simulink subsystem "rss_FaltInfoMng"  (R2023a)
settings: Solver=VariableStepAuto  StartTime=0.0  StopTime=10.0  RelTol=1e-3
undefined symbols (not defined in the file): Cdbl_tiSlwTaskSmpTi, Gbol_enFaltInfoManClr_C, Gu16_ctFaltDiaComSdlCnt_C, Gu16_ctFaltDiaFstSdlCnt_C, Gu16_ctFaltDiaSlwSdlCnt_C, Gu16_stCtlDFPMSt_C
libraries: simulink x5
settings Model: Creator=xiaoqiang.yuan  LastModifiedBy=xiaoqiang.yuan

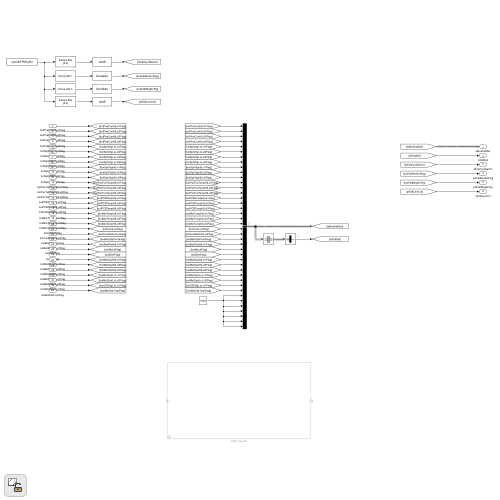
[thumbnail: Simulink's stored preview of the top-level diagram]
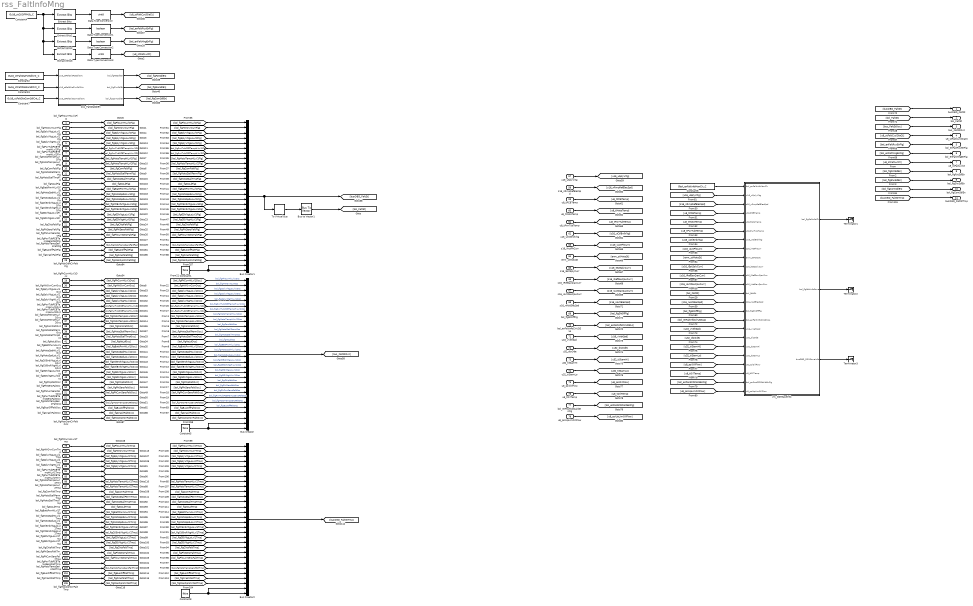
== system rss_FaltInfoMng ==
  bol_flgPhCurrHiLvl1Flg : Inport
  bol_flgHWOvrCurrFlg : Inport  Port=2
  bol_flgSplyVltgLoLvl1Flg : Inport  Port=3
  bol_flgSplyVltgLoLvl2Flg : Inport  Port=4
  bol_flgSplyVltgHiLvl1Flg : Inport  Port=5
  bol_flgPwrTubPCBTempHiLvl1Flg : Inport  Port=6
  bol_flgPwrTubPCBTempHiLvl2Flg : Inport  Port=7
  bol_flgMotoTempHiLvl1Flg : Inport  Port=8
  bol_flgMotoTempHiLvl2Flg : Inport  Port=9
  bol_flgComFaltFlg : Inport  Port=10
  bol_flgMotoStallPermFlg : Inport  Port=11
  bol_flgMotoStallTmpFlg : Inport  Port=12
  bol_flgNoLdFlg : Inport  Port=13
  bol_flgBattPwrHiLvl1Flg : Inport  Port=14
  bol_flgMotoSpdHiLvl1Flg : Inport  Port=15
  bol_flgMotoSpdLoLvl1Flg : Inport  Port=16
  bol_flgCtlBrdVltgLoLvl1Flg : Inport  Port=17
  bol_flgCtlBrdVltgHiLvl1Flg : Inport  Port=18
  bol_flgGDVltgLoLvl1Flg : Inport  Port=19
  bol_flgGDVltgHiLvl1Flg : Inport  Port=20
  bol_flgChipFaltFlg : Inport  Port=21
  bol_flgPhiSensFaltFlg : Inport  Port=22
  bol_flgPhCurrSensFaltFlg : Inport  Port=23
  bol_flgPwrTubPCBTempSensFaltFlg : Inport  Port=24
  bol_flgMotoTempSensFaltFlg : Inport  Port=25
  bol_flgBusOffFaltFlg : Inport  Port=26
  bol_flgCrashFaltFlg : Inport  Port=27
  bol_flgMosOpnCirFaltFlg : Inport  Port=28
  bol_flgPhCurrHiLvl1Occ : Inport  Port=29
  bol_flgHWOvrCurrOcc : Inport  Port=30
  bol_flgSplyVltgLoLvl1Occ : Inport  Port=31
  bol_flgSplyVltgLoLvl2Occ : Inport  Port=32
  bol_flgSplyVltgHiLvl1Occ : Inport  Port=33
  bol_flgPwrTubPCBTempHiLvl1Occ : Inport  Port=34
  bol_flgPwrTubPCBTempHiLvl2Occ : Inport  Port=35
  bol_flgMotoTempHiLvl1Occ : Inport  Port=36
  bol_flgMotoTempHiLvl2Occ : Inport  Port=37
  bol_flgComFaltOcc : Inport  Port=38
  bol_flgMotoStallPermOcc : Inport  Port=39
  bol_flgMotoStallTmpOcc : Inport  Port=40
  bol_flgNoLdOcc : Inport  Port=41
  bol_flgBattPwrHiLvl1Occ : Inport  Port=42
  bol_flgMotoSpdHiLvl1Occ : Inport  Port=43
  bol_flgMotoSpdLoLvl1Occ : Inport  Port=44
  bol_flgCtlBrdVltgLoLvl1Occ : Inport  Port=45
  bol_flgCtlBrdVltgHiLvl1Occ : Inport  Port=46
  bol_flgGDVltgLoLvl1Occ : Inport  Port=47
  bol_flgGDVltgHiLvl1Occ : Inport  Port=48
  bol_flgChipFaltOcc : Inport  Port=49
  bol_flgPhiSensFaltOcc : Inport  Port=50
  bol_flgPhCurrSensFaltOcc : Inport  Port=51
  bol_flgPwrTubPCBTempSensFaltOcc : Inport  Port=52
  bol_flgMotoTempSensFaltOcc : Inport  Port=53
  bol_flgBusOffFaltOcc : Inport  Port=54
  bol_flgCrashFaltOcc : Inport  Port=55
  bol_flgMosOpnCirFaltOcc : Inport  Port=56
  u16_uSplyVltg : Inport  Port=57  OutDataTypeStr=dt_Standardize_u16p15b0
  s16_nRmpRefElecSpd : Inport  Port=58  OutDataTypeStr=dt_Standardize_s16p15b0
  u8_tPCBTemp : Inport  Port=59  OutDataTypeStr=dt_Temp_u8p0bn40
  u8_tMotoTemp : Inport  Port=60  OutDataTypeStr=dt_Temp_u8p0bn40
  u8_tPwrTubTemp : Inport  Port=61  OutDataTypeStr=dt_Temp_u8p0bn40
  u16_uCtlBrdVltg : Inport  Port=62  OutDataTypeStr=dt_Standardize_u16p15b0
  s16_iActPhCurr : Inport  Port=63  OutDataTypeStr=dt_Standardize_s16p15b0
  enm_stMotoSt : Inport  Port=64  OutDataTypeStr=Enum: ENM_MOTO_STATUS
  s16_iEstSplyCurr : Inport  Port=65  OutDataTypeStr=dt_Standardize_s16p15b0
  s16_iRefDaxQaxCurr : Inport  Port=66  OutDataTypeStr=dt_Standardize_s16p15b0
  s16_iActDaxQaxCurr : Inport  Port=67  OutDataTypeStr=dt_Standardize_s16p15b0
  s16_nActElecSpd : Inport  Port=68  OutDataTypeStr=dt_Standardize_s16p15b0
  bol_flgShOffFlg : Inport  Port=69  OutDataTypeStr=boolean
  bol_enFaltInfoClrUDS14 : Inport  Port=70  OutDataTypeStr=boolean
  u16_vVehSpd : Inport  Port=71  OutDataTypeStr=fixdt(0,16,10^-2,0)
  u32_disOde : Inport  Port=72  OutDataTypeStr=fixdt(0,32,10^-1,0)
  u32_tiStamHi : Inport  Port=73  OutDataTypeStr=uint32
  u32_tiStamLo : Inport  Port=74  OutDataTypeStr=uint32
  u8_psiOilFlow : Inport  Port=75  OutDataTypeStr=fixdt(0,8,5^-1,0)
  u8_tOilTemp : Inport  Port=76  OutDataTypeStr=dt_Temp_u8p0bn40
  bol_enPosSCDCalibEnFlg : Inport  Port=77  OutDataTypeStr=boolean
  u8_psiUpLimOilFlow : Inport  Port=78  OutDataTypeStr=fixdt(0,8,5^-1,0)
  bol_flgPhCurrHiLvl1Tmp : Inport  Port=79  OutDataTypeStr=boolean
  bol_flgHWOvrCurrTmp : Inport  Port=80  OutDataTypeStr=boolean
  bol_flgSplyVltgLoLvl1Tmp : Inport  Port=81  OutDataTypeStr=boolean
  bol_flgSplyVltgLoLvl2Tmp : Inport  Port=82  OutDataTypeStr=boolean
  bol_flgSplyVltgHiLvl1Tmp : Inport  Port=83  OutDataTypeStr=boolean
  bol_flgPwrTubPCBTempHiLvl1Tmp : Inport  Port=84  OutDataTypeStr=boolean
  bol_flgPwrTubPCBTempHiLvl2Tmp : Inport  Port=85  OutDataTypeStr=boolean
  bol_flgMotoTempHiLvl1Tmp : Inport  Port=86  OutDataTypeStr=boolean
  bol_flgMotoTempHiLvl2Tmp : Inport  Port=87  OutDataTypeStr=boolean
  bol_flgComFaltTmp : Inport  Port=88  OutDataTypeStr=boolean
  bol_flgMotoStallPermTmp : Inport  Port=89  OutDataTypeStr=boolean
  bol_flgMotoStallTmpTmp : Inport  Port=90  OutDataTypeStr=boolean
  bol_flgNoLdTmp : Inport  Port=91  OutDataTypeStr=boolean
  bol_flgBattPwrHiLvl1Tmp : Inport  Port=92  OutDataTypeStr=boolean
  bol_flgMotoSpdHiLvl1Tmp : Inport  Port=93  OutDataTypeStr=boolean
  bol_flgMotoSpdLoLvl1Tmp : Inport  Port=94  OutDataTypeStr=boolean
  bol_flgCtlBrdVltgLoLvl1Tmp : Inport  Port=95  OutDataTypeStr=boolean
  bol_flgCtlBrdVltgHiLvl1Tmp : Inport  Port=96  OutDataTypeStr=boolean
  bol_flgGDVltgLoLvl1Tmp : Inport  Port=97  OutDataTypeStr=boolean
  bol_flgGDVltgHiLvl1Tmp : Inport  Port=98  OutDataTypeStr=boolean
  bol_flgChipFaltTmp : Inport  Port=99  OutDataTypeStr=boolean
  bol_flgPhiSensFaltTmp : Inport  Port=100  OutDataTypeStr=boolean
  bol_flgPhCurrSensFaltTmp : Inport  Port=101  OutDataTypeStr=boolean
  bol_flgPwrTubPCBTempSensFaltTmp : Inport  Port=102  OutDataTypeStr=boolean
  bol_flgMotoTempSensFaltTmp : Inport  Port=103  OutDataTypeStr=boolean
  bol_flgBusOffFaltTmp : Inport  Port=104  OutDataTypeStr=boolean
  bol_flgCrashFaltTmp : Inport  Port=105  OutDataTypeStr=boolean
  bol_flgMosOpnCirFaltTmp : Inport  Port=106  OutDataTypeStr=boolean
  Bus Creator : BusCreator  Inputs=30
  Bus Creator1 : BusCreator  Inputs=30  OutDataTypeStr=Bus: BUS_OBD_FALT_STS  NonVirtualBus=on
      settings: InheritFromInputs=off
  Bus Creator2 : BusCreator  Inputs=30  OutDataTypeStr=Bus: BUS_OBD_FALT_STS_TMP  NonVirtualBus=on
      settings: InheritFromInputs=off
  Bus to Vector1 : BusToVector
  Constant1 : Constant  Value=false  OutDataTypeStr=boolean
  Constant2 : Constant  Value=Gu16_ctFaltDiaFstSdlCnt_C
  Constant3 : Constant  Value=Gu16_ctFaltDiaSlwSdlCnt_C
  Constant4 : Constant  Value=Gu16_stCtlDFPMSt_C
  Constant5 : Constant  Value=false  OutDataTypeStr=boolean
  Constant6 : Constant  Value=Gbol_enFaltInfoManClr_C
  Constant7 : Constant  Value=Gu16_ctFaltDiaComSdlCnt_C
  Constant8 : Constant  Value=false  OutDataTypeStr=boolean
  Data Type Conversion : DataTypeConversion  OutDataTypeStr=uint8  SaturateOnIntegerOverflow=off  RndMeth=Floor
  Data Type Conversion1 : DataTypeConversion  OutDataTypeStr=boolean  SaturateOnIntegerOverflow=off  RndMeth=Floor
  Data Type Conversion2 : DataTypeConversion  OutDataTypeStr=boolean  SaturateOnIntegerOverflow=off  RndMeth=Floor
  Data Type Conversion3 : DataTypeConversion  OutDataTypeStr=uint8  SaturateOnIntegerOverflow=off  RndMeth=Floor
  Extract Bits : simulink/Logic and Bit Operations/Extract Bits  bitsToExtract=Range of bits  numBits=8  bitIdxRange=[4 7]  outScalingMode=Treat bit field as an integer
  Extract Bits1 : simulink/Logic and Bit Operations/Extract Bits  bitsToExtract=Range of bits  numBits=8  bitIdxRange=0  outScalingMode=Treat bit field as an integer
  Extract Bits2 : simulink/Logic and Bit Operations/Extract Bits  bitsToExtract=Range of bits  numBits=8  bitIdxRange=3  outScalingMode=Treat bit field as an integer
  Extract Bits3 : simulink/Logic and Bit Operations/Extract Bits  bitsToExtract=Range of bits  numBits=8  bitIdxRange=[1 2]  outScalingMode=Treat bit field as an integer
  Terminator1 : Terminator
  Terminator2 : Terminator
  Terminator3 : Terminator
  To Virtual Bus : SignalConversion  ConversionOutput=Virtual bus  OverrideOpt=off
  sss_FaltDiaSdlEn : Subsystem
  vrs_DSMSaveInfo : Subsystem  Variant=on  VariantControlMode=label  VariantControl=Choice  LabelModeActiveChoice=DSMSaveInfoNoNeed
  busOBD_FaltSt : Outport  OutDataTypeStr=Bus: BUS_OBD_FALT_STS
  bol_FaltSt : Outport  Port=2  OutDataTypeStr=boolean
  bus_FaltStOcc : Outport  Port=3
  u8_stFaltCyclDiaCt : Outport  Port=4  OutDataTypeStr=uint8
  bol_enFaltRcvEnFlg : Outport  Port=5  OutDataTypeStr=boolean
  bol_enFaltMngEnFlg : Outport  Port=6  OutDataTypeStr=boolean
  u8_stFaltLvlCt : Outport  Port=7  OutDataTypeStr=uint8
  bol_flgFstSdlEn : Outport  Port=8  OutDataTypeStr=boolean
  bol_flgSlwSdlEn : Outport  Port=9  OutDataTypeStr=boolean
  bol_flgComSdlEn : Outport  Port=10  OutDataTypeStr=boolean
  busOBD_FaltStTmp : Outport  Port=11  OutDataTypeStr=Bus: BUS_OBD_FALT_STS_TMP
  wires:
  Bus Creator1/1 -> [busOBD_FaltSt], To Virtual Bus/1
  [bol_flgMotoStallPermFlg] -> Bus Creator1/11
  [bol_flgPhiSensFaltFlg] -> Bus Creator1/22
  Constant1/1 -> Bus Creator1/30, Bus Creator1/29
  [bol_flgNoLdFlg] -> Bus Creator1/13
  [bol_flgMotoTempHiLvl1Flg] -> Bus Creator1/8
  [bol_flgMotoSpdHiLvl1Flg] -> Bus Creator1/15
  [bol_flgMotoStallTmpFlg] -> Bus Creator1/12
  [bol_flgCtlBrdVltgLoLvl1Flg] -> Bus Creator1/17
  [bol_flgCtlBrdVltgHiLvl1Flg] -> Bus Creator1/18
  [bol_flgPhCurrHiLvl1Flg] -> Bus Creator1/1
  [bol_flgGDVltgLoLvl1Flg] -> Bus Creator1/19
  [bol_flgComFaltFlg] -> Bus Creator1/10
  [bol_flgBattPwrHiLvl1Flg] -> Bus Creator1/14
  [bol_flgSplyVltgHiLvl1Flg] -> Bus Creator1/5
  [bol_flgPhCurrSensFaltFlg] -> Bus Creator1/23
  [bol_flgMotoTempHiLvl2Flg] -> Bus Creator1/9
  [bol_flgPwrTubPCBTempHiLvl1Flg] -> Bus Creator1/6
  [bol_flgMotoTempSensFaltFlg] -> Bus Creator1/25
  [bol_flgHWOvrCurrFlg] -> Bus Creator1/2
  [bol_flgPwrTubPCBTempSensFaltFlg] -> Bus Creator1/24
  [bol_flgSplyVltgLoLvl2Flg] -> Bus Creator1/4
  [bol_flgPwrTubPCBTempHiLvl2Flg] -> Bus Creator1/7
  [bol_flgMotoSpdLoLvl1Flg] -> Bus Creator1/16
  [bol_flgGDVltgHiLvl1Flg] -> Bus Creator1/20
  [bol_flgChipFaltFlg] -> Bus Creator1/21
  Extract Bits1/1 -> Data Type Conversion1/1
  Extract Bits/1 -> Data Type Conversion/1
  Extract Bits2/1 -> Data Type Conversion2/1
  Data Type Conversion2/1 -> [bol_enFaltMngEnFlg]
  Data Type Conversion/1 -> [u8_stFaltCyclDiaCt]
  Data Type Conversion1/1 -> [bol_enFaltRcvEnFlg]
  [u8_stFaltCyclDiaCt] -> u8_stFaltCyclDiaCt/1
  [bol_enFaltRcvEnFlg] -> bol_enFaltRcvEnFlg/1
  [bol_enFaltMngEnFlg] -> bol_enFaltMngEnFlg/1
  [busOBD_FaltSt] -> busOBD_FaltSt/1
  [bol_FaltSt] -> bol_FaltSt/1
  Bus to Vector1/1 -> [bol_FaltSt]
  [bol_flgSplyVltgLoLvl1Flg] -> Bus Creator1/3
  Extract Bits3/1 -> Data Type Conversion3/1
  Constant4/1 -> Extract Bits/1, Extract Bits1/1, Extract Bits2/1, Extract Bits3/1
  Data Type Conversion3/1 -> [u8_stFaltLvlCt]
  [u8_stFaltLvlCt] -> u8_stFaltLvlCt/1
  bol_flgPhCurrHiLvl1Flg/1 -> [bol_flgPhCurrHiLvl1Flg]
  bol_flgHWOvrCurrFlg/1 -> [bol_flgHWOvrCurrFlg]
  bol_flgSplyVltgLoLvl1Flg/1 -> [bol_flgSplyVltgLoLvl1Flg]
  bol_flgSplyVltgLoLvl2Flg/1 -> [bol_flgSplyVltgLoLvl2Flg]
  bol_flgSplyVltgHiLvl1Flg/1 -> [bol_flgSplyVltgHiLvl1Flg]
  bol_flgPwrTubPCBTempHiLvl1Flg/1 -> [bol_flgPwrTubPCBTempHiLvl1Flg]
  bol_flgPwrTubPCBTempHiLvl2Flg/1 -> [bol_flgPwrTubPCBTempHiLvl2Flg]
  bol_flgMotoTempHiLvl1Flg/1 -> [bol_flgMotoTempHiLvl1Flg]
  bol_flgMotoTempHiLvl2Flg/1 -> [bol_flgMotoTempHiLvl2Flg]
  bol_flgComFaltFlg/1 -> [bol_flgComFaltFlg]
  bol_flgMotoStallPermFlg/1 -> [bol_flgMotoStallPermFlg]
  bol_flgMotoStallTmpFlg/1 -> [bol_flgMotoStallTmpFlg]
  bol_flgNoLdFlg/1 -> [bol_flgNoLdFlg]
  bol_flgBattPwrHiLvl1Flg/1 -> [bol_flgBattPwrHiLvl1Flg]
  bol_flgMotoSpdHiLvl1Flg/1 -> [bol_flgMotoSpdHiLvl1Flg]
  bol_flgMotoSpdLoLvl1Flg/1 -> [bol_flgMotoSpdLoLvl1Flg]
  bol_flgCtlBrdVltgLoLvl1Flg/1 -> [bol_flgCtlBrdVltgLoLvl1Flg]
  bol_flgCtlBrdVltgHiLvl1Flg/1 -> [bol_flgCtlBrdVltgHiLvl1Flg]
  bol_flgGDVltgLoLvl1Flg/1 -> [bol_flgGDVltgLoLvl1Flg]
  bol_flgGDVltgHiLvl1Flg/1 -> [bol_flgGDVltgHiLvl1Flg]
  bol_flgChipFaltFlg/1 -> [bol_flgChipFaltFlg]
  bol_flgPhiSensFaltFlg/1 -> [bol_flgPhiSensFaltFlg]
  bol_flgPhCurrSensFaltFlg/1 -> [bol_flgPhCurrSensFaltFlg]
  bol_flgPwrTubPCBTempSensFaltFlg/1 -> [bol_flgPwrTubPCBTempSensFaltFlg]
  bol_flgMotoTempSensFaltFlg/1 -> [bol_flgMotoTempSensFaltFlg]
  Constant3/1 -> sss_FaltDiaSdlEn/2(u16_ctFaltDiaSlwSdlCnt)
  Constant2/1 -> sss_FaltDiaSdlEn/1(u16_ctFaltDiaFstSdlCnt)
  sss_FaltDiaSdlEn/1(bol_flgFstSdlEn) -> [bol_flgFstSdlEn]
  sss_FaltDiaSdlEn/2(bol_flgSlwSdlEn) -> [bol_flgSlwSdlEn]
  [bol_flgFstSdlEn] -> bol_flgFstSdlEn/1
  [bol_flgSlwSdlEn] -> bol_flgSlwSdlEn/1
  Constant5/1 -> Bus Creator/30, Bus Creator/29
  [bol_flgSplyVltgLoLvl1Occ] -> Bus Creator/3  "bol_flgSplyVltgLoLvl1Occ"
  [bol_flgMotoTempSensFaltOcc] -> Bus Creator/25  "bol_flgMotoTempSensFaltOcc"
  bol_flgPwrTubPCBTempHiLvl2Occ/1 -> [bol_flgPwrTubPCBTempHiLvl2Occ]
  bol_flgMotoTempSensFaltOcc/1 -> [bol_flgMotoTempSensFaltOcc]
  bol_flgPhiSensFaltOcc/1 -> [bol_flgPhiSensFaltOcc]
  [bol_flgSplyVltgLoLvl2Occ] -> Bus Creator/4  "bol_flgSplyVltgLoLvl2Occ"
  bol_flgPhCurrSensFaltOcc/1 -> [bol_flgPhCurrSensFaltOcc]
  [bol_flgGDVltgLoLvl1Occ] -> Bus Creator/19  "bol_flgGDVltgLoLvl1Occ"
  bol_flgMotoTempHiLvl2Occ/1 -> [bol_flgMotoTempHiLvl2Occ]
  bol_flgGDVltgLoLvl1Occ/1 -> [bol_flgGDVltgLoLvl1Occ]
  bol_flgMotoStallTmpOcc/1 -> [bol_flgMotoStallTmpOcc]
  bol_flgGDVltgHiLvl1Occ/1 -> [bol_flgGDVltgHiLvl1Occ]
  bol_flgCtlBrdVltgLoLvl1Occ/1 -> [bol_flgCtlBrdVltgLoLvl1Occ]
  bol_flgComFaltOcc/1 -> [bol_flgComFaltOcc]
  bol_flgMotoSpdHiLvl1Occ/1 -> [bol_flgMotoSpdHiLvl1Occ]
  bol_flgPhCurrHiLvl1Occ/1 -> [bol_flgPhCurrHiLvl1Occ]
  bol_flgBattPwrHiLvl1Occ/1 -> [bol_flgBattPwrHiLvl1Occ]
  bol_flgSplyVltgHiLvl1Occ/1 -> [bol_flgSplyVltgHiLvl1Occ]
  bol_flgMotoSpdLoLvl1Occ/1 -> [bol_flgMotoSpdLoLvl1Occ]
  bol_flgSplyVltgLoLvl1Occ/1 -> [bol_flgSplyVltgLoLvl1Occ]
  bol_flgHWOvrCurrOcc/1 -> [bol_flgHWOvrCurrOcc]
  bol_flgPwrTubPCBTempHiLvl1Occ/1 -> [bol_flgPwrTubPCBTempHiLvl1Occ]
  bol_flgSplyVltgLoLvl2Occ/1 -> [bol_flgSplyVltgLoLvl2Occ]
  [bol_flgPwrTubPCBTempSensFaltOcc] -> Bus Creator/24  "bol_flgPwrTubPCBTempSensFaltOcc"
  [bol_flgSplyVltgHiLvl1Occ] -> Bus Creator/5  "bol_flgSplyVltgHiLvl1Occ"
  [bol_flgMotoSpdHiLvl1Occ] -> Bus Creator/15  "bol_flgMotoSpdHiLvl1Occ"
  [bol_flgPwrTubPCBTempHiLvl2Occ] -> Bus Creator/7  "bol_flgPwrTubPCBTempHiLvl2Occ"
  bol_flgMotoStallPermOcc/1 -> [bol_flgMotoStallPermOcc]
  [bol_flgComFaltOcc] -> Bus Creator/10  "bol_flgComFaltOcc"
  [bol_flgPwrTubPCBTempHiLvl1Occ] -> Bus Creator/6  "bol_flgPwrTubPCBTempHiLvl1Occ"
  [bol_flgHWOvrCurrOcc] -> Bus Creator/2  "bol_flgHWOvrCurrOcc"
  [bol_flgChipFaltOcc] -> Bus Creator/21  "bol_flgChipFaltOcc"
  [bol_flgMotoTempHiLvl2Occ] -> Bus Creator/9  "bol_flgMotoTempHiLvl2Occ"
  [bol_flgMotoTempHiLvl1Occ] -> Bus Creator/8  "bol_flgMotoTempHiLvl1Occ"
  [bol_flgPhiSensFaltOcc] -> Bus Creator/22  "bol_flgPhiSensFaltOcc"
  bol_flgChipFaltOcc/1 -> [bol_flgChipFaltOcc]
  [bol_flgPhCurrHiLvl1Occ] -> Bus Creator/1  "bol_flgPhCurrHiLvl1Occ"
  [bol_flgNoLdOcc] -> Bus Creator/13  "bol_flgNoLdOcc"
  bol_flgCtlBrdVltgHiLvl1Occ/1 -> [bol_flgCtlBrdVltgHiLvl1Occ]
  bol_flgPwrTubPCBTempSensFaltOcc/1 -> [bol_flgPwrTubPCBTempSensFaltOcc]
  [bol_flgBattPwrHiLvl1Occ] -> Bus Creator/14  "bol_flgBattPwrHiLvl1Occ"
  [bol_flgCtlBrdVltgLoLvl1Occ] -> Bus Creator/17  "bol_flgCtlBrdVltgLoLvl1Occ"
  [bol_flgMotoSpdLoLvl1Occ] -> Bus Creator/16  "bol_flgMotoSpdLoLvl1Occ"
  bol_flgMotoTempHiLvl1Occ/1 -> [bol_flgMotoTempHiLvl1Occ]
  [bol_flgMotoStallTmpOcc] -> Bus Creator/12  "bol_flgMotoStallTmpOcc"
  [bol_flgCtlBrdVltgHiLvl1Occ] -> Bus Creator/18  "bol_flgCtlBrdVltgHiLvl1Occ"
  [bol_flgPhCurrSensFaltOcc] -> Bus Creator/23  "bol_flgPhCurrSensFaltOcc"
  bol_flgNoLdOcc/1 -> [bol_flgNoLdOcc]
  [bol_flgMotoStallPermOcc] -> Bus Creator/11  "bol_flgMotoStallPermOcc"
  [bol_flgGDVltgHiLvl1Occ] -> Bus Creator/20  "bol_flgGDVltgHiLvl1Occ"
  Bus Creator/1 -> [bus_FaltStOcc]
  [bus_FaltStOcc] -> bus_FaltStOcc/1
  To Virtual Bus/1 -> Bus to Vector1/1
  u16_uSplyVltg/1 -> [u16_uSplyVltg]
  s16_nRmpRefElecSpd/1 -> [s16_nRmpRefElecSpd]
  u8_tPCBTemp/1 -> [u8_tPCBTemp]
  u8_tMotoTemp/1 -> [u8_tMotoTemp]
  u8_tPwrTubTemp/1 -> [u8_tPwrTubTemp]
  u16_uCtlBrdVltg/1 -> [u16_uCtlBrdVltg]
  s16_iActPhCurr/1 -> [s16_iActPhCurr]
  enm_stMotoSt/1 -> [enm_stMotoSt]
  s16_iEstSplyCurr/1 -> [s16_iEstSplyCurr]
  s16_iRefDaxQaxCurr/1 -> [s16_iRefDaxQaxCurr]
  s16_iActDaxQaxCurr/1 -> [s16_iActDaxQaxCurr]
  s16_nActElecSpd/1 -> [s16_nActElecSpd]
  bol_flgShOffFlg/1 -> [bol_flgShOffFlg]
  Constant6/1 -> vrs_DSMSaveInfo/1(bol_enFaltInfoManClr)
  [u16_uSplyVltg] -> vrs_DSMSaveInfo/2(u16_uSplyVltg)
  [s16_nRmpRefElecSpd] -> vrs_DSMSaveInfo/3(s16_nRmpRefElecSpd)
  [u8_tPCBTemp] -> vrs_DSMSaveInfo/4(u8_tPCBTemp)
  [u8_tMotoTemp] -> vrs_DSMSaveInfo/5(u8_tMotoTemp)
  [u8_tPwrTubTemp] -> vrs_DSMSaveInfo/6(u8_tPwrTubTemp)
  [u16_uCtlBrdVltg] -> vrs_DSMSaveInfo/7(u16_uCtlBrdVltg)
  [s16_iActPhCurr] -> vrs_DSMSaveInfo/8(s16_iActPhCurr)
  [enm_stMotoSt] -> vrs_DSMSaveInfo/9(enm_stMotoSt)
  [s16_iEstSplyCurr] -> vrs_DSMSaveInfo/10(s16_iEstSplyCurr)
  [s16_iRefDaxQaxCurr] -> vrs_DSMSaveInfo/11(s16_iRefDaxQaxCurr)
  [s16_iActDaxQaxCurr] -> vrs_DSMSaveInfo/12(s16_iActDaxQaxCurr)
  [bol_FaltSt] -> vrs_DSMSaveInfo/13(bol_FaltSt)
  [s16_nActElecSpd] -> vrs_DSMSaveInfo/14(s16_nActElecSpd)
  [bol_flgShOffFlg] -> vrs_DSMSaveInfo/15(bol_flgShOffFlg)
  vrs_DSMSaveInfo/1(bol_flgFaltInfoClr) -> Terminator1/1
  vrs_DSMSaveInfo/2(bol_flgFaltInfoSave) -> Terminator2/1
  [bol_enFaltInfoClrUDS14] -> vrs_DSMSaveInfo/16(bol_enFaltInfoClrUDS14)
  [u16_vVehSpd] -> vrs_DSMSaveInfo/17(u16_vVehSpd)
  [u32_disOde] -> vrs_DSMSaveInfo/18(u32_disOde)
  [u32_tiStamHi] -> vrs_DSMSaveInfo/19(u32_tiStamHi)
  [u32_tiStamLo] -> vrs_DSMSaveInfo/20(u32_tiStamLo)
  [u8_psiOilFlow] -> vrs_DSMSaveInfo/21(u8_psiOilFlow)
  [u8_tOilTemp] -> vrs_DSMSaveInfo/22(u8_tOilTemp)
  [bol_enPosSCDCalibEnFlg] -> vrs_DSMSaveInfo/23(bol_enPosSCDCalibEnFlg)
  [u8_psiUpLimOilFlow] -> vrs_DSMSaveInfo/24(u8_psiUpLimOilFlow)
  bol_enFaltInfoClrUDS14/1 -> [bol_enFaltInfoClrUDS14]
  u16_vVehSpd/1 -> [u16_vVehSpd]
  u32_disOde/1 -> [u32_disOde]
  u32_tiStamHi/1 -> [u32_tiStamHi]
  u32_tiStamLo/1 -> [u32_tiStamLo]
  u8_psiOilFlow/1 -> [u8_psiOilFlow]
  u8_tOilTemp/1 -> [u8_tOilTemp]
  bol_enPosSCDCalibEnFlg/1 -> [bol_enPosSCDCalibEnFlg]
  u8_psiUpLimOilFlow/1 -> [u8_psiUpLimOilFlow]
  [bol_flgBusOffFaltFlg] -> Bus Creator1/26
  bol_flgBusOffFaltFlg/1 -> [bol_flgBusOffFaltFlg]
  [bol_flgBusOffFaltOcc] -> Bus Creator/26  "bol_flgBusOffFaltOcc"
  bol_flgBusOffFaltOcc/1 -> [bol_flgBusOffFaltOcc]
  Constant7/1 -> sss_FaltDiaSdlEn/3(u16_ctFaltDiaComSdlCnt)
  sss_FaltDiaSdlEn/3(bol_flgComSdlEn) -> [bol_flgComSdlEn]
  [bol_flgComSdlEn] -> bol_flgComSdlEn/1
  vrs_DSMSaveInfo/3(busOBD_DSMSaveInfo) -> Terminator3/1
  bol_flgCrashFaltFlg/1 -> [bol_flgCrashFaltFlg]
  [bol_flgCrashFaltFlg] -> Bus Creator1/27
  bol_flgCrashFaltOcc/1 -> [bol_flgCrashFaltOcc]
  [bol_flgCrashFaltOcc] -> Bus Creator/27
  [bol_flgMosOpnCirFaltFlg] -> Bus Creator1/28
  bol_flgMosOpnCirFaltFlg/1 -> [bol_flgMosOpnCirFaltFlg]
  [bol_flgMosOpnCirFaltOcc] -> Bus Creator/28
  bol_flgMosOpnCirFaltOcc/1 -> [bol_flgMosOpnCirFaltOcc]
  bol_flgMosOpnCirFaltTmp/1 -> [bol_flgMosOpnCirFaltTmp]
  bol_flgChipFaltTmp/1 -> [bol_flgChipFaltTmp]
  bol_flgPhCurrHiLvl1Tmp/1 -> [bol_flgPhCurrHiLvl1Tmp]
  bol_flgMotoStallTmpTmp/1 -> [bol_flgMotoStallTmpTmp]
  bol_flgPwrTubPCBTempSensFaltTmp/1 -> [bol_flgPwrTubPCBTempSensFaltTmp]
  bol_flgMotoTempHiLvl1Tmp/1 -> [bol_flgMotoTempHiLvl1Tmp]
  bol_flgMotoSpdLoLvl1Tmp/1 -> [bol_flgMotoSpdLoLvl1Tmp]
  bol_flgPwrTubPCBTempHiLvl1Tmp/1 -> [bol_flgPwrTubPCBTempHiLvl1Tmp]
  bol_flgSplyVltgLoLvl2Tmp/1 -> [bol_flgSplyVltgLoLvl2Tmp]
  bol_flgHWOvrCurrTmp/1 -> [bol_flgHWOvrCurrTmp]
  bol_flgPhiSensFaltTmp/1 -> [bol_flgPhiSensFaltTmp]
  bol_flgMotoSpdHiLvl1Tmp/1 -> [bol_flgMotoSpdHiLvl1Tmp]
  bol_flgGDVltgHiLvl1Tmp/1 -> [bol_flgGDVltgHiLvl1Tmp]
  bol_flgMotoTempHiLvl2Tmp/1 -> [bol_flgMotoTempHiLvl2Tmp]
  Bus Creator2/1 -> [busOBD_FaltStTmp]
  bol_flgComFaltTmp/1 -> [bol_flgComFaltTmp]
  bol_flgPhCurrSensFaltTmp/1 -> [bol_flgPhCurrSensFaltTmp]
  bol_flgPwrTubPCBTempHiLvl2Tmp/1 -> [bol_flgPwrTubPCBTempHiLvl2Tmp]
  bol_flgSplyVltgHiLvl1Tmp/1 -> [bol_flgSplyVltgHiLvl1Tmp]
  bol_flgMotoTempSensFaltTmp/1 -> [bol_flgMotoTempSensFaltTmp]
  bol_flgCtlBrdVltgHiLvl1Tmp/1 -> [bol_flgCtlBrdVltgHiLvl1Tmp]
  bol_flgCrashFaltTmp/1 -> [bol_flgCrashFaltTmp]
  bol_flgBattPwrHiLvl1Tmp/1 -> [bol_flgBattPwrHiLvl1Tmp]
  bol_flgGDVltgLoLvl1Tmp/1 -> [bol_flgGDVltgLoLvl1Tmp]
  bol_flgMotoStallPermTmp/1 -> [bol_flgMotoStallPermTmp]
  bol_flgSplyVltgLoLvl1Tmp/1 -> [bol_flgSplyVltgLoLvl1Tmp]
  bol_flgCtlBrdVltgLoLvl1Tmp/1 -> [bol_flgCtlBrdVltgLoLvl1Tmp]
  bol_flgBusOffFaltTmp/1 -> [bol_flgBusOffFaltTmp]
  bol_flgNoLdTmp/1 -> [bol_flgNoLdTmp]
  [busOBD_FaltStTmp] -> busOBD_FaltStTmp/1
  Constant8/1 -> Bus Creator2/30, Bus Creator2/29
  [bol_flgPhCurrHiLvl1Tmp] -> Bus Creator2/1
  [bol_flgHWOvrCurrTmp] -> Bus Creator2/2
  [bol_flgSplyVltgLoLvl1Tmp] -> Bus Creator2/3
  [bol_flgSplyVltgLoLvl2Tmp] -> Bus Creator2/4
  [bol_flgSplyVltgHiLvl1Tmp] -> Bus Creator2/5
  [bol_flgPwrTubPCBTempHiLvl1Tmp] -> Bus Creator2/6
  [bol_flgPwrTubPCBTempHiLvl2Tmp] -> Bus Creator2/7
  [bol_flgMotoTempHiLvl1Tmp] -> Bus Creator2/8
  [bol_flgMotoTempHiLvl2Tmp] -> Bus Creator2/9
  [bol_flgComFaltTmp] -> Bus Creator2/10
  [bol_flgMotoStallPermTmp] -> Bus Creator2/11
  [bol_flgMotoStallTmpTmp] -> Bus Creator2/12
  [bol_flgNoLdTmp] -> Bus Creator2/13
  [bol_flgBattPwrHiLvl1Tmp] -> Bus Creator2/14
  [bol_flgMotoSpdHiLvl1Tmp] -> Bus Creator2/15
  [bol_flgMotoSpdLoLvl1Tmp] -> Bus Creator2/16
  [bol_flgCtlBrdVltgLoLvl1Tmp] -> Bus Creator2/17
  [bol_flgCtlBrdVltgHiLvl1Tmp] -> Bus Creator2/18
  [bol_flgGDVltgLoLvl1Tmp] -> Bus Creator2/19
  [bol_flgGDVltgHiLvl1Tmp] -> Bus Creator2/20
  [bol_flgChipFaltTmp] -> Bus Creator2/21
  [bol_flgPhiSensFaltTmp] -> Bus Creator2/22
  [bol_flgPhCurrSensFaltTmp] -> Bus Creator2/23
  [bol_flgPwrTubPCBTempSensFaltTmp] -> Bus Creator2/24
  [bol_flgMotoTempSensFaltTmp] -> Bus Creator2/25
  [bol_flgBusOffFaltTmp] -> Bus Creator2/26
  [bol_flgCrashFaltTmp] -> Bus Creator2/27
  [bol_flgMosOpnCirFaltTmp] -> Bus Creator2/28

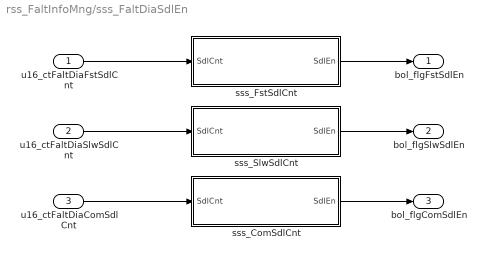
== system rss_FaltInfoMng/sss_FaltDiaSdlEn ==
  u16_ctFaltDiaFstSdlCnt : Inport
  u16_ctFaltDiaSlwSdlCnt : Inport  Port=2
  u16_ctFaltDiaComSdlCnt : Inport  Port=3
  sss_ComSdlCnt : Subsystem  RTWFcnName=counter_10  RTWFileName=MotorControlLib
      settings: RTWFcnNameOpts=User specified  RTWFileNameOpts=User specified
  sss_FstSdlCnt : Subsystem  RTWFcnName=counter_10  RTWFileName=MotorControlLib
      settings: RTWFcnNameOpts=User specified  RTWFileNameOpts=User specified
  sss_SlwSdlCnt : Subsystem  RTWFcnName=counter_10  RTWFileName=MotorControlLib
      settings: RTWFcnNameOpts=User specified  RTWFileNameOpts=User specified
  bol_flgFstSdlEn : Outport
  bol_flgSlwSdlEn : Outport  Port=2
  bol_flgComSdlEn : Outport  Port=3
  wires:
  sss_ComSdlCnt/1(SdlEn) -> bol_flgComSdlEn/1
  u16_ctFaltDiaComSdlCnt/1 -> sss_ComSdlCnt/1(SdlCnt)
  u16_ctFaltDiaSlwSdlCnt/1 -> sss_SlwSdlCnt/1(SdlCnt)
  sss_SlwSdlCnt/1(SdlEn) -> bol_flgSlwSdlEn/1
  sss_FstSdlCnt/1(SdlEn) -> bol_flgFstSdlEn/1
  u16_ctFaltDiaFstSdlCnt/1 -> sss_FstSdlCnt/1(SdlCnt)

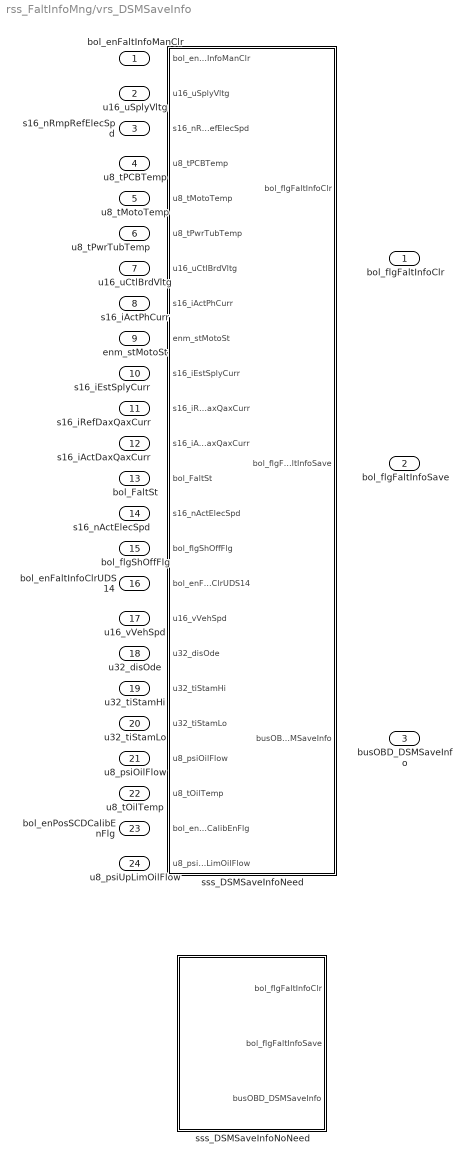
== system rss_FaltInfoMng/vrs_DSMSaveInfo ==
  bol_enFaltInfoManClr : Inport
  u16_uSplyVltg : Inport  Port=2
  s16_nRmpRefElecSpd : Inport  Port=3
  u8_tPCBTemp : Inport  Port=4
  u8_tMotoTemp : Inport  Port=5
  u8_tPwrTubTemp : Inport  Port=6
  u16_uCtlBrdVltg : Inport  Port=7
  s16_iActPhCurr : Inport  Port=8
  enm_stMotoSt : Inport  Port=9
  s16_iEstSplyCurr : Inport  Port=10
  s16_iRefDaxQaxCurr : Inport  Port=11
  s16_iActDaxQaxCurr : Inport  Port=12
  bol_FaltSt : Inport  Port=13
  s16_nActElecSpd : Inport  Port=14
  bol_flgShOffFlg : Inport  Port=15
  bol_enFaltInfoClrUDS14 : Inport  Port=16
  u16_vVehSpd : Inport  Port=17
  u32_disOde : Inport  Port=18
  u32_tiStamHi : Inport  Port=19
  u32_tiStamLo : Inport  Port=20
  u8_psiOilFlow : Inport  Port=21
  u8_tOilTemp : Inport  Port=22
  bol_enPosSCDCalibEnFlg : Inport  Port=23
  u8_psiUpLimOilFlow : Inport  Port=24
  sss_DSMSaveInfoNeed : Subsystem  RTWFcnName=OBD_DSM_SaveInf  RTWFileName=OBD_DSM  VariantControl=DSMSaveInfoNeed
      settings: RTWSystemCode=Nonreusable function  RTWFcnNameOpts=User specified  RTWFileNameOpts=User specified
  sss_DSMSaveInfoNoNeed : Subsystem  VariantControl=DSMSaveInfoNoNeed
  bol_flgFaltInfoClr : Outport
  bol_flgFaltInfoSave : Outport  Port=2
  busOBD_DSMSaveInfo : Outport  Port=3

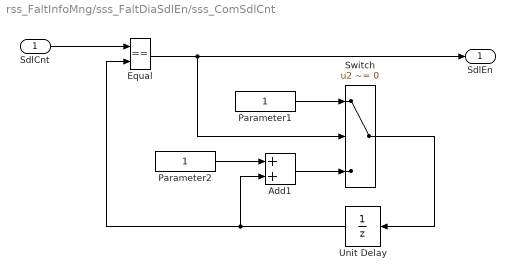
== system rss_FaltInfoMng/sss_FaltDiaSdlEn/sss_ComSdlCnt ==
  SdlCnt : Inport
      settings: AttributesFormatString=%<Description>cnt_max=n-1 n为总次数
  Add1 : Sum  OutDataTypeStr=Inherit: Same as first input
  Equal : RelationalOperator  Operator===  OutDataTypeStr=boolean
  Parameter1 : Constant  OutDataTypeStr=uint16  SampleTime=-1
      settings: AttributesFormatString=SampleTime=%<SampleTime>
  Parameter2 : Constant  OutDataTypeStr=uint16  SampleTime=-1
      settings: AttributesFormatString=SampleTime=%<SampleTime>
  Switch : Switch  Criteria=u2 ~= 0  SaturateOnIntegerOverflow=off  OutDataTypeStr=Inherit: Same as first input
      settings: AttributesFormatString=InputSameDT=%<InputSameDT>
  Unit Delay : UnitDelay  InitialCondition=1  SampleTime=-1  HasFrameUpgradeWarning=on
  SdlEn : Outport
  wires:
  SdlCnt/1 -> Equal/1
  Parameter2/1 -> Add1/1
  Equal/1 -> Switch/2, SdlEn/1
  Unit Delay/1 -> Add1/2, Equal/2
  Parameter1/1 -> Switch/1
  Switch/1 -> Unit Delay/1
  Add1/1 -> Switch/3

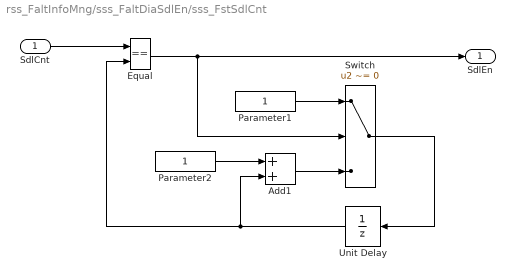
== system rss_FaltInfoMng/sss_FaltDiaSdlEn/sss_FstSdlCnt ==
  SdlCnt : Inport
      settings: AttributesFormatString=%<Description>cnt_max=n-1 n为总次数
  Add1 : Sum  OutDataTypeStr=Inherit: Same as first input
  Equal : RelationalOperator  Operator===  OutDataTypeStr=boolean
  Parameter1 : Constant  OutDataTypeStr=uint16  SampleTime=-1
      settings: AttributesFormatString=SampleTime=%<SampleTime>
  Parameter2 : Constant  OutDataTypeStr=uint16  SampleTime=-1
      settings: AttributesFormatString=SampleTime=%<SampleTime>
  Switch : Switch  Criteria=u2 ~= 0  SaturateOnIntegerOverflow=off  OutDataTypeStr=Inherit: Same as first input
      settings: AttributesFormatString=InputSameDT=%<InputSameDT>
  Unit Delay : UnitDelay  InitialCondition=1  SampleTime=-1  HasFrameUpgradeWarning=on
  SdlEn : Outport
  wires:
  Add1/1 -> Switch/3
  Switch/1 -> Unit Delay/1
  Parameter1/1 -> Switch/1
  Unit Delay/1 -> Equal/2, Add1/2
  Equal/1 -> SdlEn/1, Switch/2
  Parameter2/1 -> Add1/1
  SdlCnt/1 -> Equal/1

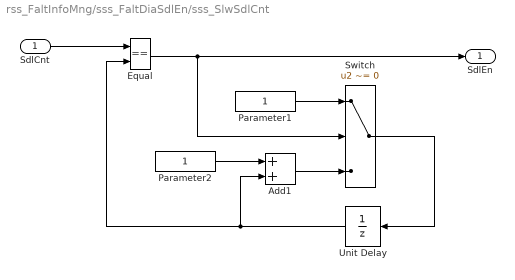
== system rss_FaltInfoMng/sss_FaltDiaSdlEn/sss_SlwSdlCnt ==
  SdlCnt : Inport
      settings: AttributesFormatString=%<Description>cnt_max=n-1 n为总次数
  Add1 : Sum  OutDataTypeStr=Inherit: Same as first input
  Equal : RelationalOperator  Operator===  OutDataTypeStr=boolean
  Parameter1 : Constant  OutDataTypeStr=uint16  SampleTime=-1
      settings: AttributesFormatString=SampleTime=%<SampleTime>
  Parameter2 : Constant  OutDataTypeStr=uint16  SampleTime=-1
      settings: AttributesFormatString=SampleTime=%<SampleTime>
  Switch : Switch  Criteria=u2 ~= 0  SaturateOnIntegerOverflow=off  OutDataTypeStr=Inherit: Same as first input
      settings: AttributesFormatString=InputSameDT=%<InputSameDT>
  Unit Delay : UnitDelay  InitialCondition=1  SampleTime=-1  HasFrameUpgradeWarning=on
  SdlEn : Outport
  wires:
  SdlCnt/1 -> Equal/1
  Parameter2/1 -> Add1/1
  Equal/1 -> Switch/2, SdlEn/1
  Unit Delay/1 -> Add1/2, Equal/2
  Parameter1/1 -> Switch/1
  Switch/1 -> Unit Delay/1
  Add1/1 -> Switch/3

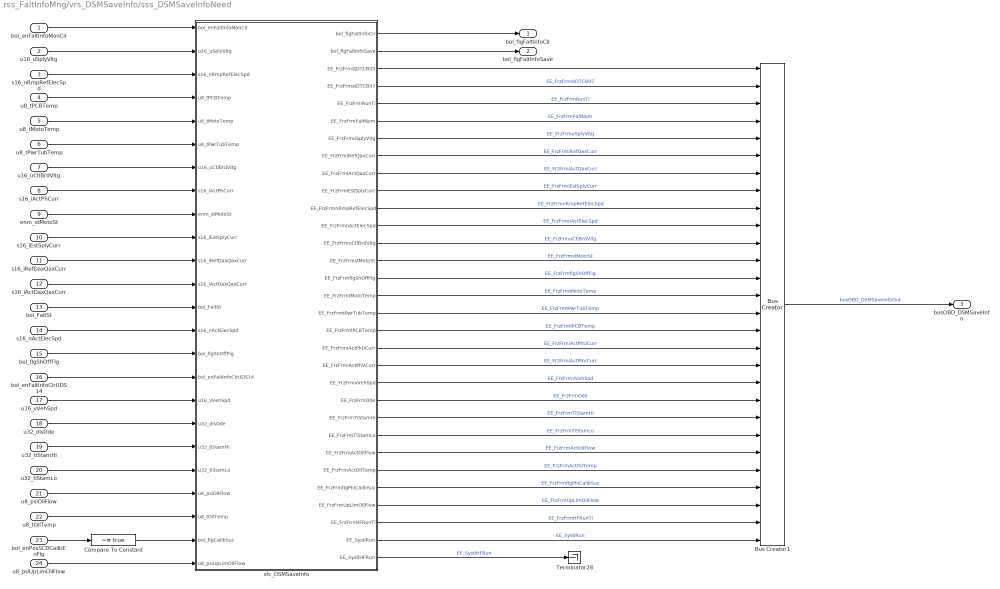
== system rss_FaltInfoMng/vrs_DSMSaveInfo/sss_DSMSaveInfoNeed ==
  bol_enFaltInfoManClr : Inport
  u16_uSplyVltg : Inport  Port=2
  s16_nRmpRefElecSpd : Inport  Port=3
  u8_tPCBTemp : Inport  Port=4
  u8_tMotoTemp : Inport  Port=5
  u8_tPwrTubTemp : Inport  Port=6
  u16_uCtlBrdVltg : Inport  Port=7
  s16_iActPhCurr : Inport  Port=8
  enm_stMotoSt : Inport  Port=9
  s16_iEstSplyCurr : Inport  Port=10
  s16_iRefDaxQaxCurr : Inport  Port=11
  s16_iActDaxQaxCurr : Inport  Port=12
  bol_FaltSt : Inport  Port=13
  s16_nActElecSpd : Inport  Port=14
  bol_flgShOffFlg : Inport  Port=15
  bol_enFaltInfoClrUDS14 : Inport  Port=16
  u16_vVehSpd : Inport  Port=17
  u32_disOde : Inport  Port=18
  u32_tiStamHi : Inport  Port=19
  u32_tiStamLo : Inport  Port=20
  u8_psiOilFlow : Inport  Port=21
  u8_tOilTemp : Inport  Port=22
  bol_enPosSCDCalibEnFlg : Inport  Port=23
  u8_psiUpLimOilFlow : Inport  Port=24
  Bus Creator1 : BusCreator  Inputs=28  OutDataTypeStr=Bus: BUS_OBD_DSM_SAVE_INFO  NonVirtualBus=on
      settings: InheritFromInputs=off
  Compare To Constant : simulink/Logic and Bit Operations/Compare To Constant  relop=~=  const=true  OutDataTypeStr=boolean
  Terminator28 : Terminator
  sfc_DSMSaveInfo : Stateflow chart  TreatAsAtomicUnit=on
  bol_flgFaltInfoClr : Outport
  bol_flgFaltInfoSave : Outport  Port=2
  busOBD_DSMSaveInfo : Outport  Port=3  OutDataTypeStr=Bus: BUS_OBD_DSM_SAVE_INFO  SampleTime=round(double(Cdbl_tiSlwTaskSmpTi),4)
  wires:
  sfc_DSMSaveInfo/3(EE_FrzFrmstDTCBit3) -> Bus Creator1/1
  Bus Creator1/1 -> busOBD_DSMSaveInfo/1  "busOBD_DSMSaveInfoOut"
  Compare To Constant/1 -> sfc_DSMSaveInfo/23(bol_flgCalibSuc)
  sfc_DSMSaveInfo/29(EE_FrzFrmHFRunTi) -> Bus Creator1/27  "EE_FrzFrmHFRunTi"
  u8_psiUpLimOilFlow/1 -> sfc_DSMSaveInfo/24(u8_psiUpLimOilFlow)
  bol_enPosSCDCalibEnFlg/1 -> Compare To Constant/1
  u8_tOilTemp/1 -> sfc_DSMSaveInfo/22(u8_tOilTemp)
  u8_psiOilFlow/1 -> sfc_DSMSaveInfo/21(u8_psiOilFlow)
  u32_tiStamLo/1 -> sfc_DSMSaveInfo/20(u32_tiStamLo)
  u32_tiStamHi/1 -> sfc_DSMSaveInfo/19(u32_tiStamHi)
  u32_disOde/1 -> sfc_DSMSaveInfo/18(u32_disOde)
  u16_vVehSpd/1 -> sfc_DSMSaveInfo/17(u16_vVehSpd)
  bol_enFaltInfoClrUDS14/1 -> sfc_DSMSaveInfo/16(bol_enFaltInfoClrUDS14)
  bol_flgShOffFlg/1 -> sfc_DSMSaveInfo/15(bol_flgShOffFlg)
  s16_nActElecSpd/1 -> sfc_DSMSaveInfo/14(s16_nActElecSpd)
  bol_FaltSt/1 -> sfc_DSMSaveInfo/13(bol_FaltSt)
  s16_iActDaxQaxCurr/1 -> sfc_DSMSaveInfo/12(s16_iActDaxQaxCurr)
  s16_iRefDaxQaxCurr/1 -> sfc_DSMSaveInfo/11(s16_iRefDaxQaxCurr)
  s16_iEstSplyCurr/1 -> sfc_DSMSaveInfo/10(s16_iEstSplyCurr)
  enm_stMotoSt/1 -> sfc_DSMSaveInfo/9(enm_stMotoSt)
  s16_iActPhCurr/1 -> sfc_DSMSaveInfo/8(s16_iActPhCurr)
  u16_uCtlBrdVltg/1 -> sfc_DSMSaveInfo/7(u16_uCtlBrdVltg)
  u8_tPwrTubTemp/1 -> sfc_DSMSaveInfo/6(u8_tPwrTubTemp)
  u8_tMotoTemp/1 -> sfc_DSMSaveInfo/5(u8_tMotoTemp)
  u8_tPCBTemp/1 -> sfc_DSMSaveInfo/4(u8_tPCBTemp)
  s16_nRmpRefElecSpd/1 -> sfc_DSMSaveInfo/3(s16_nRmpRefElecSpd)
  u16_uSplyVltg/1 -> sfc_DSMSaveInfo/2(u16_uSplyVltg)
  bol_enFaltInfoManClr/1 -> sfc_DSMSaveInfo/1(bol_enFaltInfoManClr)
  sfc_DSMSaveInfo/31(EE_SystiHFRun) -> Terminator28/1  "EE_SystiHFRun"
  sfc_DSMSaveInfo/30(EE_SystiRun) -> Bus Creator1/28  "EE_SystiRun"
  sfc_DSMSaveInfo/25(EE_FrzFrmActOilFlow) -> Bus Creator1/23  "EE_FrzFrmActOilFlow"
  sfc_DSMSaveInfo/18(EE_FrzFrmtPCBTemp) -> Bus Creator1/16  "EE_FrzFrmtPCBTemp"
  sfc_DSMSaveInfo/28(EE_FrzFrmUpLimOilFlow) -> Bus Creator1/26  "EE_FrzFrmUpLimOilFlow"
  sfc_DSMSaveInfo/27(EE_FrzFrmflgPhiCalibSuc) -> Bus Creator1/25  "EE_FrzFrmflgPhiCalibSuc"
  sfc_DSMSaveInfo/26(EE_FrzFrmActOilTemp) -> Bus Creator1/24  "EE_FrzFrmActOilTemp"
  sfc_DSMSaveInfo/6(EE_FrzFrmFaltNum) -> Bus Creator1/4  "EE_FrzFrmFaltNum"
  sfc_DSMSaveInfo/1(bol_flgFaltInfoClr) -> bol_flgFaltInfoClr/1
  sfc_DSMSaveInfo/2(bol_flgFaltInfoSave) -> bol_flgFaltInfoSave/1
  sfc_DSMSaveInfo/16(EE_FrzFrmtMotoTemp) -> Bus Creator1/14  "EE_FrzFrmtMotoTemp"
  sfc_DSMSaveInfo/14(EE_FrzFrmstMotoSt) -> Bus Creator1/12  "EE_FrzFrmstMotoSt"
  sfc_DSMSaveInfo/22(EE_FrzFrmOde) -> Bus Creator1/20  "EE_FrzFrmOde"
  sfc_DSMSaveInfo/17(EE_FrzFrmtPwrTubTemp) -> Bus Creator1/15  "EE_FrzFrmtPwrTubTemp"
  sfc_DSMSaveInfo/24(EE_FrzFrmTiStamLo) -> Bus Creator1/22  "EE_FrzFrmTiStamLo"
  sfc_DSMSaveInfo/23(EE_FrzFrmTiStamHi) -> Bus Creator1/21  "EE_FrzFrmTiStamHi"
  sfc_DSMSaveInfo/15(EE_FrzFrmflgShOffFlg) -> Bus Creator1/13  "EE_FrzFrmflgShOffFlg"
  sfc_DSMSaveInfo/4(EE_FrzFrmstDTCBit7) -> Bus Creator1/2  "EE_FrzFrmstDTCBit7"
  sfc_DSMSaveInfo/5(EE_FrzFrmRunTi) -> Bus Creator1/3  "EE_FrzFrmRunTi"
  sfc_DSMSaveInfo/12(EE_FrzFrmnActElecSpd) -> Bus Creator1/10  "EE_FrzFrmnActElecSpd"
  sfc_DSMSaveInfo/11(EE_FrzFrmnRmpRefElecSpd) -> Bus Creator1/9  "EE_FrzFrmnRmpRefElecSpd"
  sfc_DSMSaveInfo/7(EE_FrzFrmuSplyVltg) -> Bus Creator1/5  "EE_FrzFrmuSplyVltg"
  sfc_DSMSaveInfo/13(EE_FrzFrmuCtlBrdVltg) -> Bus Creator1/11  "EE_FrzFrmuCtlBrdVltg"
  sfc_DSMSaveInfo/21(EE_FrzFrmvVehSpd) -> Bus Creator1/19  "EE_FrzFrmvVehSpd"
  sfc_DSMSaveInfo/20(EE_FrzFrmiActPhVCurr) -> Bus Creator1/18  "EE_FrzFrmiActPhVCurr"
  sfc_DSMSaveInfo/19(EE_FrzFrmiActPhUCurr) -> Bus Creator1/17  "EE_FrzFrmiActPhUCurr"
  sfc_DSMSaveInfo/8(EE_FrzFrmiRefQaxCurr) -> Bus Creator1/6  "EE_FrzFrmiRefQaxCurr"
  sfc_DSMSaveInfo/10(EE_FrzFrmiEstSplyCurr) -> Bus Creator1/8  "EE_FrzFrmiEstSplyCurr"
  sfc_DSMSaveInfo/9(EE_FrzFrmiActQaxCurr) -> Bus Creator1/7  "EE_FrzFrmiActQaxCurr"

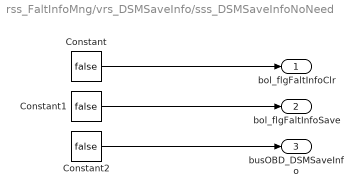
== system rss_FaltInfoMng/vrs_DSMSaveInfo/sss_DSMSaveInfoNoNeed ==
  Constant : Constant  Value=false  OutDataTypeStr=boolean
  Constant1 : Constant  Value=false  OutDataTypeStr=boolean
  Constant2 : Constant  Value=false  OutDataTypeStr=boolean
  bol_flgFaltInfoClr : Outport
  bol_flgFaltInfoSave : Outport  Port=2
  busOBD_DSMSaveInfo : Outport  Port=3
  wires:
  Constant2/1 -> busOBD_DSMSaveInfo/1
  Constant1/1 -> bol_flgFaltInfoSave/1
  Constant/1 -> bol_flgFaltInfoClr/1

== stateflow chart rss_FaltInfoMng/vrs_DSMSaveInfo/sss_DSMSaveInfoNeed/sfc_DSMSaveInfo ==
  state SysTiRun [function]
    (default) -> (junction 144)
    (junction 144) -> (junction 146) : {EE_SystiHFRun++;
        | timer++;}
    (junction 146) -> (junction 148) [order 1] : [timer>=uint16(100)]
    (junction 146) -> (junction 152) [order 2]
    (junction 148) -> (junction 150) : {EE_SystiRun=EE_SystiRun+uint32(1);
        | EE_SystiHFRun=uint16(0);
        | timer=uint16(0);}
    (junction 150) -> (junction 152)
    (junction 152) -> (junction 155)
  state SaveFreezeInfo [function]
    (default) -> (junction 19)
    (junction 19) -> (junction 60) : {EE_FrzFrmRunTi[k]=EE_SystiRun;
        | EE_FrzFrmHFRunTi[k]=EE_SystiHFRun;
        | EE_FrzFrmuSplyVltg[k]=u16_uSplyVltg;
        | EE_FrzFrmiRefQaxCurr[k]=s16_iRefDaxQaxCurr[1];
        | EE_FrzFrmiActQaxCurr[k]=s16_iActDaxQaxCurr[1];
        | EE_FrzFrmiEstSplyCurr[k]=s16_iEstSplyCurr;
        | EE_FrzFrmnRmpRefElecSpd[k]=s16_nRmpRefElecSpd;
        | EE_FrzFrmnActElecSpd[k]=s16_nActElecSpd;
        | EE_FrzFrmuCtlBrdVltg[k]=u16_uCtlBrdVltg;
        | EE_FrzFrmstMotoSt[k]=enm_stMotoSt;
        | EE_FrzFrmflgShOffFlg[k]=bol_flgShOffFlg;
        | EE_FrzFrmtPCBTemp[k]=u8_tPCBTemp;
        | EE_FrzFrmtMotoTemp[k]=u8_tMotoTemp;
        | EE_FrzFrmtPwrTubTemp[k]=u8_tPwrTubTemp;
        | EE_FrzFrmiActPhUCurr[k]=s16_iActPhCurr[0];
        | EE_FrzFrmiActPhVCurr[k]=s16_iActPhCurr[1];
        | EE_FrzFrmvVehSpd[k]=u16_vVehSpd;
        | EE_FrzFrmOde[k]=u32_disOde;
        | EE_FrzFrmTiStamHi[k]=u32_tiStamHi;
        | EE_FrzFrmTiStamLo[k]=u32_tiStamLo;
        | EE_FrzFrmActOilFlow[k]=u8_psiOilFlow;
        | EE_FrzFrmActOilTemp[k]=u8_tOilTemp;
        | EE_FrzFrmflgPhiCalibSuc[k]=bol_flgCalibSuc;
        | EE_FrzFrmUpLimOilFlow[k]=u8_psiUpLimOilFlow;}
  state ClearInfo [function]
    (default) -> (junction 63)
    (junction 63) -> (junction 65) : {EE_FrzFrmstDTCBit3[k]=false;
        | EE_FrzFrmstDTCBit7[k]=false;
        | EE_FrzFrmFaltNum[k]=0;
        | EE_FrzFrmRunTi[k]=0;
        | EE_FrzFrmHFRunTi[k]=0;
        | EE_FrzFrmuSplyVltg[k]=0;
        | EE_FrzFrmiRefQaxCurr[k]=0;
        | EE_FrzFrmiActQaxCurr[k]=0;
        | EE_FrzFrmiEstSplyCurr[k]=0;
        | EE_FrzFrmnRmpRefElecSpd[k]=0;
        | EE_FrzFrmnActElecSpd[k]=0;
        | EE_FrzFrmuCtlBrdVltg[k]=0;
        | EE_FrzFrmstMotoSt[k]=0;
        | EE_FrzFrmflgShOffFlg[k]=false;
        | EE_FrzFrmtPCBTemp[k]=0;
        | EE_FrzFrmtMotoTemp[k]=0;
        | EE_FrzFrmtPwrTubTemp[k]=0;
        | EE_FrzFrmiActPhUCurr[k]=0;
        | EE_FrzFrmiActPhVCurr[k]=0;
        | EE_FrzFrmvVehSpd[k]=0;
        | EE_FrzFrmOde[k]=0;
        | EE_FrzFrmTiStamHi[k]=0;
        | EE_FrzFrmTiStamLo[k]=0;
        | EE_FrzFrmActOilFlow[k]=0;
        | EE_FrzFrmActOilTemp[k]=0;
        | EE_FrzFrmflgPhiCalibSuc[k]=false;
        | EE_FrzFrmUpLimOilFlow[k]=0;}
  (default) -> (junction 1)
  (junction 1) -> (junction 3) : {SysTiRun();
      | k=uint8(0);}
  (junction 3) -> (junction 6) [order 1] : [k<uint8(30)]
  (junction 162) -> (junction 3) : {k++;}
  (junction 3) -> (junction 54) [order 2]
  (junction 6) -> (junction 8) : {EE_FrzFrmstDTCBit3[k]=bol_FaltSt[k];
      | EE_FrzFrmFaltNumInr[k] = EE_FrzFrmFaltNum[k];}
  (junction 8) -> (junction 10) [order 1] : [(bol_FaltSt[k]==true)&&(bol_FaltStLst[k]== false)]
  (junction 8) -> (junction 21) [order 2]
  (junction 10) -> (junction 29) : {bol_flgFaltInfoSave= true;}
  (junction 29) -> (junction 31) [order 1] : [EE_FrzFrmFaltNumInr[k]>=uint8(255)]
  (junction 29) -> (junction 12) [order 2] : {EE_FrzFrmFaltNumInr[k]++;}
  (junction 31) -> (junction 33) : {EE_FrzFrmFaltNumInr[k]=uint8(255);}
  (junction 21) -> (junction 23) [order 1] : [(bol_FaltSt[k]== false)&&(bol_FaltStLst[k]==true)]
  (junction 21) -> (junction 35) [order 2]
  (junction 23) -> (junction 27) : {EE_FrzFrmstDTCBit7[k]=true;
      | bol_flgFaltInfoSave=true;}
  (junction 12) -> (junction 14) [order 1] : [EE_FrzFrmFaltNumInr[k]==uint8(1)]
  (junction 12) -> (junction 48) [order 2]
  (junction 14) -> (junction 16) : {SaveFreezeInfo();}
  (junction 27) -> (junction 35)
  (junction 35) -> (junction 56)
  (junction 48) -> (junction 56)
  (junction 16) -> (junction 48)
  (junction 33) -> (junction 16)
  (junction 56) -> (junction 38) : {EE_FrzFrmFaltNum[k] = EE_FrzFrmFaltNumInr[k];}
  (junction 38) -> (junction 40) [order 1] : [(bol_enFaltInfoManClr==true)||(bol_enFaltInfoClrUDS14==true)]
  (junction 38) -> (junction 42) [order 2]
  (junction 40) -> (junction 44) : {ClearInfo();
      | bol_flgFaltInfoClr=true;}
  (junction 44) -> (junction 42)
  (junction 42) -> (junction 51) : {bol_FaltStLst[k]=bol_FaltSt[k];}
  (junction 51) -> (junction 162)
  data: bol_enFaltInfoManClr input; u16_uSplyVltg input; s16_nRmpRefElecSpd input; u8_tPCBTemp input; u8_tMotoTemp input; u8_tPwrTubTemp input; u16_uCtlBrdVltg input; s16_iActPhCurr input size=3; enm_stMotoSt input; s16_iEstSplyCurr input; s16_iRefDaxQaxCurr input size=2; s16_iActDaxQaxCurr input size=2; bol_FaltSt input size=30; s16_nActElecSpd input; bol_flgShOffFlg input; k local uint8; bol_FaltStLst local uint8 size=30; bol_flgFaltInfoClr output boolean; timer local uint16; bol_flgFaltInfoSave output boolean; EE_FrzFrmstDTCBit3 output boolean size=30; EE_FrzFrmstDTCBit7 output boolean size=30; EE_FrzFrmRunTi output uint32 size=30; EE_FrzFrmFaltNum output uint8 size=30; EE_FrzFrmuSplyVltg output dt_Standardize_u16p15b0 size=30; EE_FrzFrmiRefQaxCurr output dt_Standardize_s16p15b0 size=30; EE_FrzFrmiActQaxCurr output dt_Standardize_s16p15b0 size=30; EE_FrzFrmiEstSplyCurr output dt_Standardize_s16p15b0 size=30; EE_FrzFrmnRmpRefElecSpd output dt_Standardize_s16p15b0 size=30; EE_FrzFrmnActElecSpd output dt_Standardize_s16p15b0 size=30; EE_FrzFrmuCtlBrdVltg output dt_Standardize_u16p15b0 size=30; EE_FrzFrmstMotoSt output Enum: ENM_MOTO_STATUS size=30; EE_FrzFrmflgShOffFlg output boolean size=30; EE_FrzFrmtMotoTemp output dt_Temp_u8p0bn40 size=30; EE_FrzFrmtPwrTubTemp output dt_Temp_u8p0bn40 size=30; EE_FrzFrmtPCBTemp output dt_Temp_u8p0bn40 size=30; EE_FrzFrmiActPhUCurr output dt_Standardize_s16p15b0 size=30; EE_FrzFrmiActPhVCurr output dt_Standardize_s16p15b0 size=30; EE_FrzFrmvVehSpd output fixdt(0,16,10^-2,0) size=30; EE_FrzFrmOde output fixdt(0,32,10^-1,0) size=30; EE_FrzFrmTiStamHi output uint32 size=30; EE_FrzFrmTiStamLo output uint32 size=30; bol_enFaltInfoClrUDS14 input boolean; EE_FrzFrmFaltNumInr local uint8 size=30; EE_FrzFrmActOilFlow output fixdt(0,8,5^-1,0) size=30; EE_FrzFrmActOilTemp output dt_Temp_u8p0bn40 size=30; EE_FrzFrmflgPhiCalibSuc output boolean size=30; EE_FrzFrmUpLimOilFlow output fixdt(0,8,5^-1,0) size=30; EE_FrzFrmHFRunTi output uint16 size=30; EE_SystiRun output uint32; EE_SystiHFRun output uint16; u16_vVehSpd input; u32_disOde input; u32_tiStamHi input; u32_tiStamLo input; u8_psiOilFlow input; u8_tOilTemp input; bol_flgCalibSuc input; u8_psiUpLimOilFlow input
